simulink model "cs"  (R2018a)
settings: Solver=FixedStepAuto  StartTime=0.0  StopTime=5  FixedStep=0.01  RelTol=1e-3
libraries: aerolibactuator x2
settings Model: Creator=Ducted Fan  LastModifiedBy=Ducted Fan

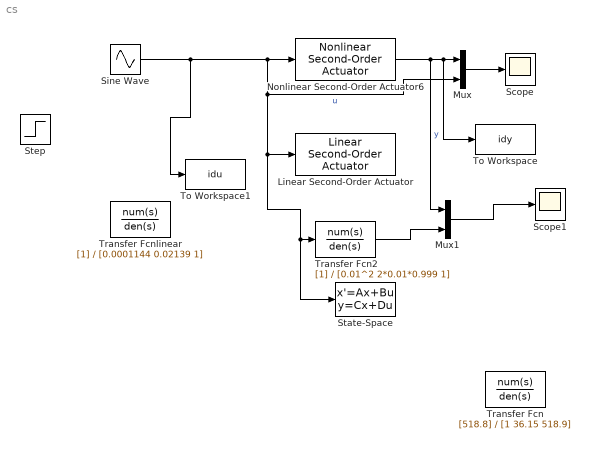
== system cs ==
  Linear Second-Order Actuator : aerolibactuator/Linear Second-Order Actuator  wn_fin=100  z_fin=1  fin_act_0=0  fin_act_vel=0
      settings: SourceProductName=Aerospace Blockset  SourceProductBaseCode=AE
  Mux : Mux  Inputs=2
  Mux1 : Mux  Inputs=2
  Nonlinear Second-Order Actuator6 : aerolibactuator/Nonlinear Second-Order Actuator  wn_fin=100  z_fin=1  fin_max=60*pi/180  fin_min=-60*pi/180  fin_maxrate=380*pi/180  fin_act_0=0  fin_act_vel=0
      settings: SourceProductName=Aerospace Blockset  SourceProductBaseCode=AE
  Scope : Scope
  Scope1 : Scope
  Sine Wave : Sin  SineType=Sample based  Samples=50  SampleTime=0.01
  State-Space : StateSpace  A=[0 1;-1/0.01^2 -2*0.9999/0.01]  B=[0;1/0.01^2]  C=[1 0]  D=0  InitialCondition=0
  Step : Step  SampleTime=0
  To Workspace : ToWorkspace  VariableName=idy  SaveFormat=Timeseries  SampleTime=-1
  To Workspace1 : ToWorkspace  VariableName=idu  SaveFormat=Timeseries  SampleTime=-1
  Transfer Fcn : TransferFcn  Numerator=[518.8]  Denominator=[1 36.15 518.9]
  Transfer Fcn2 : TransferFcn  Denominator=[0.01^2 2*0.01*0.999 1]
  Transfer Fcnlinear : TransferFcn  Denominator=[0.0001144 0.02139 1]
  wires:
  Sine Wave/1 -> State-Space/1, Transfer Fcn2/1, Linear Second-Order Actuator/1, Mux/2, Nonlinear Second-Order Actuator6/1, To Workspace1/1  "u"
  Nonlinear Second-Order Actuator6/1 -> Mux1/1, Mux/1, To Workspace/1  "y"
  Mux/1 -> Scope/1
  Mux1/1 -> Scope1/1
  Transfer Fcn2/1 -> Mux1/2
